simulink library "GTPR_Library"  (R2021a)
settings: Solver=VariableStepAuto  StartTime=0.0  StopTime=10.0  RelTol=1e-3
values from neighbouring files (symbols this model uses):
  aA = 0.5    [SimMechanics_GTPR_OpenLoop_CircularMotion_VS_ClosedLoop.m]
  aB = 0.5    [SimMechanics_GTPR_OpenLoop_CircularMotion_VS_ClosedLoop.m]
  aC = 0.5    [SimMechanics_GTPR_OpenLoop_CircularMotion_VS_ClosedLoop.m]
  alphaAB = deg2rad(120)    [SimMechanics_GTPR_OpenLoop_CircularMotion_VS_ClosedLoop.m]
  alphaAC = deg2rad(240)    [SimMechanics_GTPR_OpenLoop_CircularMotion_VS_ClosedLoop.m]
  eA = 0.28    [SimMechanics_GTPR_OpenLoop_CircularMotion_VS_ClosedLoop.m]
  eB = 0.28    [SimMechanics_GTPR_OpenLoop_CircularMotion_VS_ClosedLoop.m]
  eC = 0.28    [SimMechanics_GTPR_OpenLoop_CircularMotion_VS_ClosedLoop.m]
  g = -9.81    [SimMechanics_GTPR_OpenLoop_CircularMotion_VS_ClosedLoop.m]
  ILA = zeros(3)    [SimMechanics_GTPR_OpenLoop_CircularMotion_VS_ClosedLoop.m]
  IlA = zeros(3)    [SimMechanics_GTPR_OpenLoop_CircularMotion_VS_ClosedLoop.m]
  ILB = zeros(3)    [SimMechanics_GTPR_OpenLoop_CircularMotion_VS_ClosedLoop.m]
  IlB = zeros(3)    [SimMechanics_GTPR_OpenLoop_CircularMotion_VS_ClosedLoop.m]
  ILC = zeros(3)    [SimMechanics_GTPR_OpenLoop_CircularMotion_VS_ClosedLoop.m]
  IlC = zeros(3)    [SimMechanics_GTPR_OpenLoop_CircularMotion_VS_ClosedLoop.m]
  LA = 0.57    [SimMechanics_GTPR_OpenLoop_CircularMotion_VS_ClosedLoop.m]
  lA = 0.9    [SimMechanics_GTPR_OpenLoop_CircularMotion_VS_ClosedLoop.m]
  LB = 0.57    [SimMechanics_GTPR_OpenLoop_CircularMotion_VS_ClosedLoop.m]
  lB = 0.9    [SimMechanics_GTPR_OpenLoop_CircularMotion_VS_ClosedLoop.m]
  LC = 0.57    [SimMechanics_GTPR_OpenLoop_CircularMotion_VS_ClosedLoop.m]
  lC = 0.9    [SimMechanics_GTPR_OpenLoop_CircularMotion_VS_ClosedLoop.m]
  m_unaccounted = 1e-16    [SimMechanics_GTPR_OpenLoop_CircularMotion_VS_ClosedLoop.m]
  mLA = density_upperArm*VLA    (= 1.4415197891)    [SimMechanics_GTPR_OpenLoop_CircularMotion_VS_ClosedLoop.m]
  mlA = density_LowerArm*VlA    (= 0.190851753706)    [SimMechanics_GTPR_OpenLoop_CircularMotion_VS_ClosedLoop.m]
  mLB = density_upperArm*VLB    (= 1.4415197891)    [SimMechanics_GTPR_OpenLoop_CircularMotion_VS_ClosedLoop.m]
  mlB = density_LowerArm*VlB    (= 0.190851753706)    [SimMechanics_GTPR_OpenLoop_CircularMotion_VS_ClosedLoop.m]
  mLC = density_upperArm*VLC    (= 1.4415197891)    [SimMechanics_GTPR_OpenLoop_CircularMotion_VS_ClosedLoop.m]
  mlC = density_LowerArm*VlC    (= 0.190851753706)    [SimMechanics_GTPR_OpenLoop_CircularMotion_VS_ClosedLoop.m]
  mTCP = density_workTriangle * VTCP    [SimMechanics_GTPR_OpenLoop_CircularMotion_VS_ClosedLoop.m]
undefined symbols (not defined in the file or in its folder): dq1, dq2, dq3, q1, q2, q3, X, Y, Z
libraries: sm_lib x83, $bdroot x31, nesl_utility x24
(part 1 of 8)
settings Model: Creator=szucs  LastModifiedBy=szucs

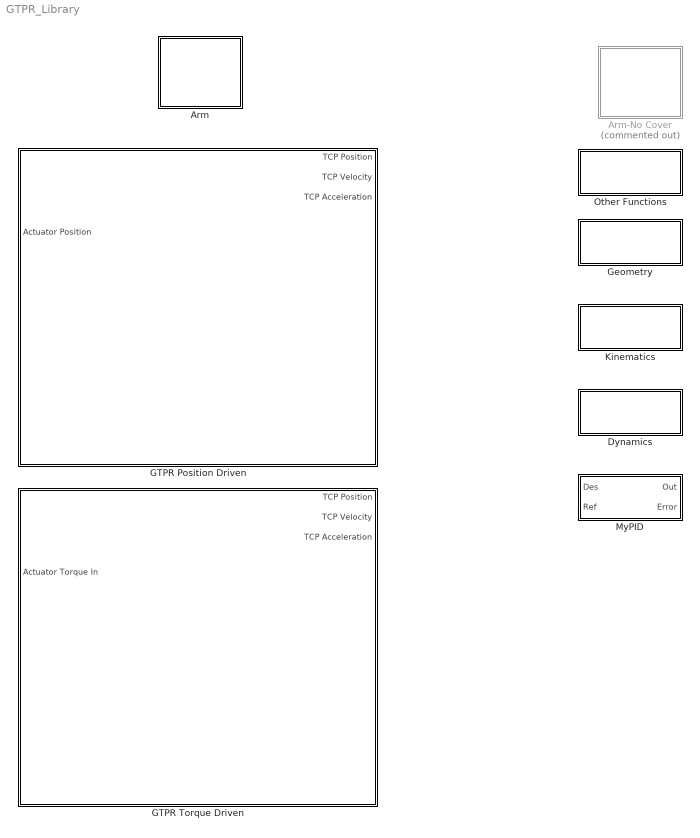
== system GTPR_Library ==
  Arm : Subsystem  mask(Delta Robot Arm){Lupper=1, RLupper=0.05, l=1, Rl=0.05, R1=0.1, L3=0.15, R2=0.05, mLupper=1, ml=1, mlink=1e-16, mTCP=0, CoverColor=[1 1 1], IL_xx=0, IL_xy=0, IL_xz=0, IL_yy=0, IL_yz=0, IL_zz=0, I_Lower_xx=0, I_Lower_xy=0, I_Lower_xz=0, I_Lower_yy=0, I_Lower_yz=0, I_Lower_zz=0}
      mask prompts: Lupper "Upper Arm Length [m]"; RLupper "Upper Arm Radius [m]"; l "Lower Arm Length [m]"; Rl "Lower Arm Radius [m]"; R1 "Joint Cover Radius [m]"; L3 "Link Length [m]"; R2 "Link Radius [m]"; mLupper "Upper Arm Mass [kg]"; ml "Lower Arm Mass [kg]"; mlink "Link Mass [kg]"; mTCP "TCP Mass [kg]"; CoverColor "Cover Color [R, G, B]"
      mask DialogControl ParameterGroupVar Prompt: Geometry
      mask DialogControl Container4 Prompt: Dimensions
      mask DialogControl Container6 Prompt: Weights
      mask DialogControl Container7 Prompt: Color
      mask DialogControl Container8 Prompt: Inertias
      mask DialogControl Container9 Prompt: Upper Arm
      mask DialogControl Container9_copy Prompt: Upper Arm
      mask Display: image(fullfile(matlabroot,'toolbox','physmod','sm','smdemos','pick_and_place_robot','images','sm_delta_robot_lib_arm.png'));
  Arm-No Cover : Subsystem  Commented=on  mask(Delta Robot Arm){Lupper=1, RLupper=0.05, l=1, Rl=0.05, R1=0.1, L3=0.15, R2=0.05, mLupper=1, ml=1, mlink=1e-16, mTCP=0, CoverColor=[1 1 1]}
      mask prompts: Lupper "Upper Arm Length [m]"; RLupper "Upper Arm Radius [m]"; l "Lower Arm Length [m]"; Rl "Lower Arm Radius [m]"; R1 "Joint Cover Radius [m]"; L3 "Link Length [m]"; R2 "Link Radius [m]"; mLupper "Upper Arm Mass [kg]"; ml "Lower Arm Mass [kg]"; mlink "Link Mass [kg]"; mTCP "TCP Mass [kg]"; CoverColor "Cover Color [R, G, B]"
      mask DialogControl ParameterGroupVar Prompt: Geometry
      mask DialogControl Container4 Prompt: Dimensions
      mask DialogControl Container6 Prompt: Weights
      mask DialogControl Container7 Prompt: Color
      mask Display: image(fullfile(matlabroot,'toolbox','physmod','sm','smdemos','pick_and_place_robot','images','sm_delta_robot_lib_arm.png'));
  Dynamics : Subsystem
  GTPR Position Driven : Subsystem  mask(Generalized Triangle Parallel Robot){LengthUpperA=LA, LengthLowerA=lA, LengthLinkA=0.1, RadiusUpperA=0.01, RadiusLowerA=0.01, RadiusLinkA=0.01, RadiusCoverA=0.02, MassUpperA=mLA, MassLowerA=mlA, MassLinkA=m_unaccounted, ColorA=[1, 0, 0], LengthUpperB=LB, LengthLowerB=lB, LengthLinkB=0.1, RadiusUpperB=0.01, RadiusLowerB=0.01, RadiusLinkB=0.01, RadiusCoverB=0.02, MassUpperB=mLB, MassLowerB=mlB, MassLinkB=m_unaccounted, ColorB=[0, 1, 0], LengthUpperC=LC, LengthLowerC=lC, LengthLinkC=0.1, RadiusUpperC=0.01, RadiusLowerC=0.01, RadiusLinkC=0.01, RadiusCoverC=0.02, MassUpperC=mLC, MassLowerC=mlC, MassLinkC=m_unaccounted, ColorC=[0, 0, 1], DistBaseA=aA, DistBaseB=aB, DistBaseC=aC, Rtop=max([aA, aB, aC]), DistWorkA=eA, DistWorkB=eB, DistWorkC=eC, MassTCP=mTCP, Rbot=max([eA, eB, eC]), NoOfSides=6, alphaAB=alphaAB, alphaAC=alphaAC}
      mask prompts: LengthUpperA "Upper Arm"; LengthLowerA "Lower Arm"; LengthLinkA "Link"; RadiusUpperA "Upper Arm"; RadiusLowerA "Lower Arm"; RadiusLinkA "Link"; RadiusCoverA "Cover"; MassUpperA "Upper Arm"; MassLowerA "Lower Arm"; MassLinkA "Link"; ColorA "Cover Color"; LengthUpperB "Upper Arm"; LengthLowerB "Lower Arm"; LengthLinkB "Link"; RadiusUpperB "Upper Arm"; RadiusLowerB "Lower Arm"; RadiusLinkB "Link"; RadiusCoverB "Cover"; MassUpperB "Upper Arm"; MassLowerB "Lower Arm"; MassLinkB "Link"; ColorB "Cover Color"; LengthUpperC "Upper Arm"; LengthLowerC "Lower Arm"; LengthLinkC "Link"; RadiusUpperC "Upper Arm"; RadiusLowerC "Lower Arm"; RadiusLinkC "Link"; RadiusCoverC "Cover"; MassUpperC "Upper Arm"; MassLowerC "Lower Arm"; MassLinkC "Link"; ColorC "Cover Color"; DistBaseA "Joint OA1 Distance [m]"; DistBaseB "Joint OB1 Distance [m]"; DistBaseC "Joint OC1 Distance [m]"; Rtop "Radius [m]"; DistWorkA "Joint TCPA3 Distance [m]"; DistWorkB "Joint TCPB3 Distance [m]"; DistWorkC "Joint TCPC3 Distance [m]"; MassTCP "Mass [kg]"; Rbot "Radius [m]"; NoOfSides "Number of Sides"; alphaAB "Angle between arms A and B [rad]"; alphaAC "Angle between arms A and C [rad]"
      mask DialogControl Container4 Prompt: Arm A
      mask DialogControl Container9 Prompt: Lengths [m]
      mask DialogControl Container10 Prompt: Radii [m]
      mask DialogControl Container11 Prompt: Masses [kg]
      mask DialogControl Container12 Prompt: Color
      mask DialogControl Container4_copy Prompt: Arm B
      mask DialogControl Container9_copy Prompt: Lengths [m]
      mask DialogControl Container10_copy Prompt: Radii [m]
      mask DialogControl Container11_copy Prompt: Masses [kg]
      mask DialogControl Container12_copy Prompt: Color
      mask DialogControl Container4_copy_copy Prompt: Arm C
      mask DialogControl Container9_copy_copy Prompt: Lengths [m]
      mask DialogControl Container10_copy_copy Prompt: Radii [m]
      mask DialogControl Container11_copy_copy Prompt: Masses [kg]
      mask DialogControl Container12_copy_copy Prompt: Color
      mask DialogControl Container25 Prompt: "Triangles" Parameters
      mask DialogControl Container27 Prompt: Base "Triangle"
      mask DialogControl Container27_copy Prompt: Work "Triangle"
  GTPR Torque Driven : Subsystem  mask(Generalized Triangle Parallel Robot){q1=q1, q2=q2, q3=q3, dq1=dq1, dq2=dq2, dq3=dq3, LengthUpperA=LA, LengthLowerA=lA, LengthLinkA=0.1, RadiusUpperA=0.01, RadiusLowerA=0.01, RadiusLinkA=0.01, RadiusCoverA=0.02, MassUpperA=mLA, MassLowerA=mlA, MassLinkA=m_unaccounted, ColorA=[1, 0, 0], IA_Upper_xx=ILA(1,1), IA_Upper_xy=ILA(1,2), IA_Upper_xz=ILA(1,3), IA_Upper_yy=ILA(2,2), IA_Upper_yz=ILA(2,3), IA_Upper_zz=ILA(3,3), IA_Lower_xx=IlA(1,1), IA_Lower_xy=IlA(1,2), IA_Lower_xz=IlA(1,3), IA_Lower_yy=IlA(2,2), IA_Lower_yz=IlA(2,3), IA_Lower_zz=IlA(3,3), LengthUpperB=LB, LengthLowerB=lB, LengthLinkB=0.1, RadiusUpperB=0.01, RadiusLowerB=0.01, RadiusLinkB=0.01, RadiusCoverB=0.02, MassUpperB=mLB, MassLowerB=mlB, MassLinkB=m_unaccounted, ColorB=[0, 1, 0], IB_Upper_xx=ILB(1,1), IB_Upper_xy=ILB(1,2), IB_Upper_xz=ILB(1,3), IB_Upper_yy=ILB(2,2), IB_Upper_yz=ILB(2,3), IB_Upper_zz=ILB(3,3), IB_Lower_xx=IlB(1,1), IB_Lower_xy=IlB(1,2), IB_Lower_xz=IlB(1,3), IB_Lower_yy=IlB(2,2), IB_Lower_yz=IlB(2,3), IB_Lower_zz=IlB(3,3), LengthUpperC=LC, LengthLowerC=lC, LengthLinkC=0.1, RadiusUpperC=0.01, RadiusLowerC=0.01, RadiusLinkC=0.01, RadiusCoverC=0.02, MassUpperC=mLC, MassLowerC=mlC, MassLinkC=m_unaccounted, ColorC=[0, 0, 1], IC_Upper_xx=ILC(1,1), IC_Upper_xy=ILC(1,2), IC_Upper_xz=ILC(1,3), IC_Upper_yy=ILC(2,2), IC_Upper_yz=ILC(2,3), IC_Upper_zz=ILC(3,3), IC_Lower_xx=IlC(1,1), IC_Lower_xy=IlC(1,2), IC_Lower_xz=IlC(1,3), IC_Lower_yy=IlC(2,2), IC_Lower_yz=IlC(2,3), IC_Lower_zz=IlC(3,3), DistBaseA=aA, DistBaseB=aB, DistBaseC=aC, Rtop=max([aA, aB, aC]), DistWorkA=eA, DistWorkB=eB, DistWorkC=eC, MassTCP=mTCP, Rbot=max([eA, eB, eC]), NoOfSides=6, alphaAB=alphaAB, alphaAC=alphaAC}
      mask prompts: q1 "Arm A Position [rad]"; q2 "Arm B Position [rad]"; q3 "Arm C Position [rad]"; dq1 "Arm A Angular Velocity [rad/s]"; dq2 "Arm B Angular Velocity [rad/s]"; dq3 "Arm C Angular Velocity [rad/s]"; LengthUpperA "Upper Arm"; LengthLowerA "Lower Arm"; LengthLinkA "Link"; RadiusUpperA "Upper Arm"; RadiusLowerA "Lower Arm"; RadiusLinkA "Link"; RadiusCoverA "Cover"; MassUpperA "Upper Arm"; MassLowerA "Lower Arm"; MassLinkA "Link"; ColorA "Cover Color"; IA_Upper_xx "I_Upper_xx"; IA_Upper_xy "I_Upper_xy"; IA_Upper_xz "I_Upper_xz"; IA_Upper_yy "I_Upper_yy"; IA_Upper_yz "I_Upper_yz"; IA_Upper_zz "I_Upper_zz"; IA_Lower_xx "I_Lower_xx"; IA_Lower_xy "I_Lower_xy"; IA_Lower_xz "I_Lower_xz"; IA_Lower_yy "I_Lower_yy"; IA_Lower_yz "I_Lower_yz"; IA_Lower_zz "I_Lower_zz"; LengthUpperB "Upper Arm"; LengthLowerB "Lower Arm"; LengthLinkB "Link"; RadiusUpperB "Upper Arm"; RadiusLowerB "Lower Arm"; RadiusLinkB "Link"; RadiusCoverB "Cover"; MassUpperB "Upper Arm"; MassLowerB "Lower Arm"; MassLinkB "Link"; ColorB "Cover Color"; IB_Upper_xx "I_Upper_xx"; IB_Upper_xy "I_Upper_xy"; IB_Upper_xz "I_Upper_xz"; IB_Upper_yy "I_Upper_yy"; IB_Upper_yz "I_Upper_yz"; IB_Upper_zz "I_Upper_zz"; IB_Lower_xx "I_Lower_xx"; IB_Lower_xy "I_Lower_xy"; IB_Lower_xz "I_Lower_xz"; IB_Lower_yy "I_Lower_yy"; IB_Lower_yz "I_Lower_yz"; IB_Lower_zz "I_Lower_zz"; LengthUpperC "Upper Arm"; LengthLowerC "Lower Arm"; LengthLinkC "Link"; RadiusUpperC "Upper Arm"; RadiusLowerC "Lower Arm"; RadiusLinkC "Link"; RadiusCoverC "Cover"; MassUpperC "Upper Arm"; MassLowerC "Lower Arm"; MassLinkC "Link"; ColorC "Cover Color"; IC_Upper_xx "I_Upper_xx"; IC_Upper_xy "I_Upper_xy"; IC_Upper_xz "I_Upper_xz"; IC_Upper_yy "I_Upper_yy"; IC_Upper_yz "I_Upper_yz"; IC_Upper_zz "I_Upper_zz"; IC_Lower_xx "I_Lower_xx"; IC_Lower_xy "I_Lower_xy"; IC_Lower_xz "I_Lower_xz"; IC_Lower_yy "I_Lower_yy"; IC_Lower_yz "I_Lower_yz"; IC_Lower_zz "I_Lower_zz"; DistBaseA "Joint OA1 Distance [m]"; DistBaseB "Joint OB1 Distance [m]"; DistBaseC "Joint OC1 Distance [m]"; Rtop "Radius [m]"; DistWorkA "Joint TCPA3 Distance [m]"; DistWorkB "Joint TCPB3 Distance [m]"; DistWorkC "Joint TCPC3 Distance [m]"; MassTCP "Mass [kg]"; Rbot "Radius [m]"; NoOfSides "Number of Sides"; alphaAB "Angle between arms A and B [rad]"; alphaAC "Angle between arms A and C [rad]"
      mask DialogControl Container32 Prompt: Initial Parameters
      mask DialogControl Container4 Prompt: Arm A
      mask DialogControl Container9 Prompt: Lengths [m]
      mask DialogControl Container10 Prompt: Radii [m]
      mask DialogControl Container11 Prompt: Masses [kg]
      mask DialogControl Container12 Prompt: Color
      mask DialogControl Container29 Prompt: Inertia Parameters
      mask DialogControl Container30 Prompt: Upper Arm
      mask DialogControl Container30_copy Prompt: Lower Arm
      mask DialogControl Container4_copy Prompt: Arm B
      mask DialogControl Container9_copy Prompt: Lengths [m]
      mask DialogControl Container10_copy Prompt: Radii [m]
      mask DialogControl Container11_copy Prompt: Masses [kg]
      mask DialogControl Container12_copy Prompt: Color
      mask DialogControl Container29_copy Prompt: Inertia Parameters
      mask DialogControl Container30_copy_copy Prompt: Upper Arm
      mask DialogControl Container30_copy_copy_copy Prompt: Lower Arm
      mask DialogControl Container4_copy_copy Prompt: Arm C
      mask DialogControl Container9_copy_copy Prompt: Lengths [m]
      mask DialogControl Container10_copy_copy Prompt: Radii [m]
      mask DialogControl Container11_copy_copy Prompt: Masses [kg]
      mask DialogControl Container12_copy_copy Prompt: Color
      mask DialogControl Container29_copy_copy Prompt: Inertia Parameters
      mask DialogControl Container30_copy_copy_copy_copy Prompt: Upper Arm
      mask DialogControl Container30_copy_copy_copy_copy_copy Prompt: Lower Arm
      mask DialogControl Container25 Prompt: "Triangles" Parameters
      mask DialogControl Container27 Prompt: Base "Triangle"
      mask DialogControl Container27_copy Prompt: Work "Triangle"
  Geometry : Subsystem
  Kinematics : Subsystem
  MyPID : Subsystem  mask{P=0, I=0, D=0}
  Other Functions : Subsystem

== system GTPR_Library/Arm ==
  Elbow Joint : sm_lib/Joints/Revolute Joint  JointMode=Normal  SenseConstraintForce=off  SenseConstraintForceX=off  SenseConstraintForceY=off  SenseConstraintForceZ=off  SenseConstraintTorque=off  SenseConstraintTorqueX=off  SenseConstraintTorqueY=off  SenseConstraintTorqueZ=off  SenseTotalForce=off  SenseTotalForceX=off  SenseTotalForceY=off  SenseTotalForceZ=off  SenseTotalTorque=off  SenseTotalTorqueX=off  SenseTotalTorqueY=off  SenseTotalTorqueZ=off  CompositeWrenchDir=FollowerOnBase  CompositeWrenchFrame=BaseFrame  EquilibriumPosition=0  EquilibriumPositionUnits=deg  SpringStiffness=0  SpringStiffnessUnits=N*m/deg  DampingCoefficient=0  DampingCoefficientUnits=N*m/(deg/s)  TorqueActuationMode=NoTorque  MotionActuationMode=ComputedMotion  SensePosition=off  SenseVelocity=off  SenseAcceleration=off  SenseTorqueForce=off  SenseLowerLimitTorqueForce=off  SenseUpperLimitTorqueForce=off  LowerLimitSpecify=off  LowerLimitBound=-90  LowerLimitBoundUnits=deg  LowerLimitStiffness=1e4  LowerLimitStiffnessUnits=N*m/deg  LowerLimitDamping=10  LowerLimitDampingUnits=N*m/(deg/s)  LowerLimitTransitionRegionWidth=0.1  LowerLimitTransitionRegionWidthUnits=deg  UpperLimitSpecify=off  UpperLimitBound=90  UpperLimitBoundUnits=deg  UpperLimitStiffness=1e4  UpperLimitStiffnessUnits=N*m/deg  UpperLimitDamping=10  UpperLimitDampingUnits=N*m/(deg/s)  UpperLimitTransitionRegionWidth=0.1  UpperLimitTransitionRegionWidthUnits=deg  PositionTargetSpecify=off  PositionTargetPriority=High  PositionTargetValue=0  PositionTargetValueUnits=deg  VelocityTargetSpecify=off  VelocityTargetPriority=High  VelocityTargetValue=0  VelocityTargetValueUnits=deg/s
  Lower Arm : Subsystem
  Upper Arm : Subsystem
  Top : PMIOPort  Side=Left
  Bot : PMIOPort  Port=2  Side=Right
  connections:
  Lower Arm/RConn1 -- Bot/RConn1
  Lower Arm/LConn1 -- Elbow Joint/RConn1
  Top/RConn1 -- Upper Arm/LConn1
  Upper Arm/RConn1 -- Elbow Joint/LConn1

== system GTPR_Library/Arm-No Cover ==
  Elbow Joint : sm_lib/Joints/Revolute Joint  JointMode=Normal  SenseConstraintForce=off  SenseConstraintForceX=off  SenseConstraintForceY=off  SenseConstraintForceZ=off  SenseConstraintTorque=off  SenseConstraintTorqueX=off  SenseConstraintTorqueY=off  SenseConstraintTorqueZ=off  SenseTotalForce=off  SenseTotalForceX=off  SenseTotalForceY=off  SenseTotalForceZ=off  SenseTotalTorque=off  SenseTotalTorqueX=off  SenseTotalTorqueY=off  SenseTotalTorqueZ=off  CompositeWrenchDir=FollowerOnBase  CompositeWrenchFrame=BaseFrame  EquilibriumPosition=0  EquilibriumPositionUnits=deg  SpringStiffness=0  SpringStiffnessUnits=N*m/deg  DampingCoefficient=0  DampingCoefficientUnits=N*m/(deg/s)  TorqueActuationMode=NoTorque  MotionActuationMode=ComputedMotion  SensePosition=off  SenseVelocity=off  SenseAcceleration=off  SenseTorqueForce=off  SenseLowerLimitTorqueForce=off  SenseUpperLimitTorqueForce=off  LowerLimitSpecify=off  LowerLimitBound=-90  LowerLimitBoundUnits=deg  LowerLimitStiffness=1e4  LowerLimitStiffnessUnits=N*m/deg  LowerLimitDamping=10  LowerLimitDampingUnits=N*m/(deg/s)  LowerLimitTransitionRegionWidth=0.1  LowerLimitTransitionRegionWidthUnits=deg  UpperLimitSpecify=off  UpperLimitBound=90  UpperLimitBoundUnits=deg  UpperLimitStiffness=1e4  UpperLimitStiffnessUnits=N*m/deg  UpperLimitDamping=10  UpperLimitDampingUnits=N*m/(deg/s)  UpperLimitTransitionRegionWidth=0.1  UpperLimitTransitionRegionWidthUnits=deg  PositionTargetSpecify=off  PositionTargetPriority=High  PositionTargetValue=0  PositionTargetValueUnits=deg  VelocityTargetSpecify=off  VelocityTargetPriority=High  VelocityTargetValue=0  VelocityTargetValueUnits=deg/s
  Lower Arm : Subsystem
  Upper Arm : Subsystem
  Top : PMIOPort  Side=Left
  Bot : PMIOPort  Port=2  Side=Right
  connections:
  Lower Arm/RConn1 -- Bot/RConn1
  Lower Arm/LConn1 -- Elbow Joint/RConn1
  Top/RConn1 -- Upper Arm/LConn1
  Upper Arm/RConn1 -- Elbow Joint/LConn1

== system GTPR_Library/Dynamics ==
  DynamicEquations : Subsystem  mask{aA=aA, aB=aB, aC=aC, alphaAB=alphaAB, alphaAC=alphaAC, LAu=LA, LBu=LB, LCu=LC, lA=lA, lB=lB, lC=lC, eA=eA, eB=eB, eC=eC, ILAu=ILA, ILBu=ILB, ILCu=ILC, IlA=IlA, IlB=IlB, IlC=IlC, g=g, mLAu=mLA, mLBu=mLB, mLCu=mLC, mlA=mlA, mlB=mlB, mlC=mlC, mTCP=mTCP}
      mask prompts: LAu "LA"; LBu "LB"; LCu "LC"; ILAu "ILA"; ILBu "ILB"; ILCu "ILC"; mLAu "mLA"; mLBu "mLB"; mLCu "mLC"
  Initialize Dynamic Equations : Subsystem  Commented=on  mask{filepath="C:\Git\PhD\Matlab\GTPR\Engine\DynamicEquations.m"}
      mask prompts: filepath "Path to "DynamicEquations.m""
  Inverse Dynamics : Subsystem  Commented=on

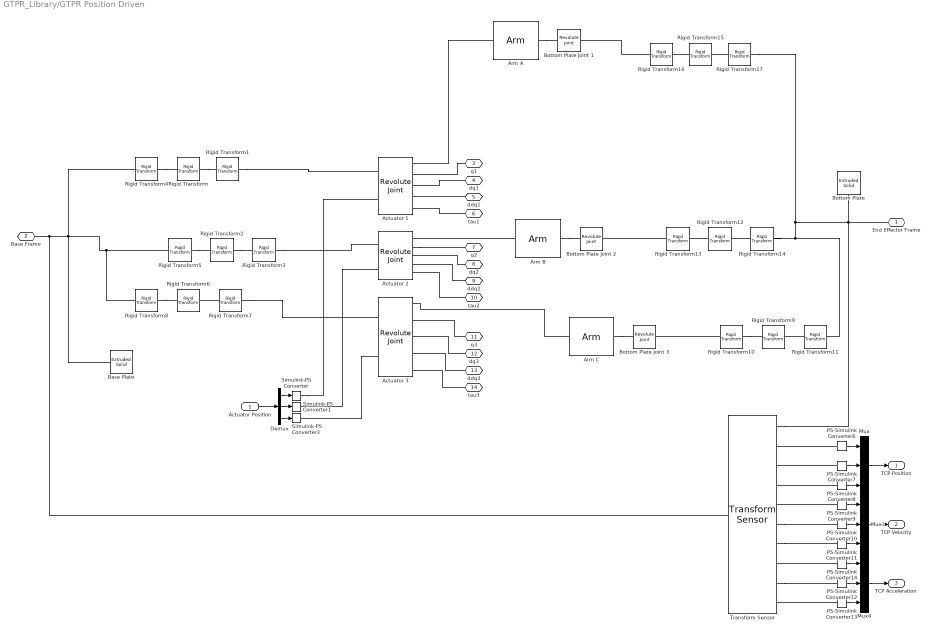
== system GTPR_Library/GTPR Position Driven ==
  Actuator Position : Inport
  Actuator 1 : sm_lib/Joints/Revolute Joint  JointMode=Normal  SenseConstraintForce=off  SenseConstraintForceX=off  SenseConstraintForceY=off  SenseConstraintForceZ=off  SenseConstraintTorque=off  SenseConstraintTorqueX=off  SenseConstraintTorqueY=off  SenseConstraintTorqueZ=off  SenseTotalForce=off  SenseTotalForceX=off  SenseTotalForceY=off  SenseTotalForceZ=off  SenseTotalTorque=off  SenseTotalTorqueX=off  SenseTotalTorqueY=off  SenseTotalTorqueZ=off  CompositeWrenchDir=FollowerOnBase  CompositeWrenchFrame=BaseFrame  EquilibriumPosition=0  EquilibriumPositionUnits=deg  SpringStiffness=0  SpringStiffnessUnits=N*m/deg  DampingCoefficient=0  DampingCoefficientUnits=N*m/(deg/s)  TorqueActuationMode=ComputedTorque  MotionActuationMode=InputMotion  SensePosition=on  SenseVelocity=on  SenseAcceleration=on  SenseTorqueForce=on  SenseLowerLimitTorqueForce=off  SenseUpperLimitTorqueForce=off  LowerLimitSpecify=off  LowerLimitBound=-10  LowerLimitBoundUnits=deg  LowerLimitStiffness=1e4  LowerLimitStiffnessUnits=N*m/deg  LowerLimitDamping=10  LowerLimitDampingUnits=N*m/(deg/s)  LowerLimitTransitionRegionWidth=0.1  LowerLimitTransitionRegionWidthUnits=deg  UpperLimitSpecify=off  UpperLimitBound=90  UpperLimitBoundUnits=deg  UpperLimitStiffness=1e4  UpperLimitStiffnessUnits=N*m/deg  UpperLimitDamping=10  UpperLimitDampingUnits=N*m/(deg/s)  UpperLimitTransitionRegionWidth=0.1  UpperLimitTransitionRegionWidthUnits=deg  PositionTargetSpecify=on  PositionTargetPriority=High  PositionTargetValue=q1  PositionTargetValueUnits=rad  VelocityTargetSpecify=on  VelocityTargetPriority=High  VelocityTargetValue=dq1  VelocityTargetValueUnits=rad/s
  Actuator 2 : sm_lib/Joints/Revolute Joint  JointMode=Normal  SenseConstraintForce=off  SenseConstraintForceX=off  SenseConstraintForceY=off  SenseConstraintForceZ=off  SenseConstraintTorque=off  SenseConstraintTorqueX=off  SenseConstraintTorqueY=off  SenseConstraintTorqueZ=off  SenseTotalForce=off  SenseTotalForceX=off  SenseTotalForceY=off  SenseTotalForceZ=off  SenseTotalTorque=off  SenseTotalTorqueX=off  SenseTotalTorqueY=off  SenseTotalTorqueZ=off  CompositeWrenchDir=FollowerOnBase  CompositeWrenchFrame=BaseFrame  EquilibriumPosition=0  EquilibriumPositionUnits=deg  SpringStiffness=0  SpringStiffnessUnits=N*m/deg  DampingCoefficient=0  DampingCoefficientUnits=N*m/(deg/s)  TorqueActuationMode=ComputedTorque  MotionActuationMode=InputMotion  SensePosition=on  SenseVelocity=on  SenseAcceleration=on  SenseTorqueForce=on  SenseLowerLimitTorqueForce=off  SenseUpperLimitTorqueForce=off  LowerLimitSpecify=off  LowerLimitBound=-10  LowerLimitBoundUnits=deg  LowerLimitStiffness=1e4  LowerLimitStiffnessUnits=N*m/deg  LowerLimitDamping=10  LowerLimitDampingUnits=N*m/(deg/s)  LowerLimitTransitionRegionWidth=0.1  LowerLimitTransitionRegionWidthUnits=deg  UpperLimitSpecify=off  UpperLimitBound=90  UpperLimitBoundUnits=deg  UpperLimitStiffness=1e4  UpperLimitStiffnessUnits=N*m/deg  UpperLimitDamping=10  UpperLimitDampingUnits=N*m/(deg/s)  UpperLimitTransitionRegionWidth=0.1  UpperLimitTransitionRegionWidthUnits=deg  PositionTargetSpecify=on  PositionTargetPriority=High  PositionTargetValue=q2  PositionTargetValueUnits=rad  VelocityTargetSpecify=on  VelocityTargetPriority=High  VelocityTargetValue=dq2  VelocityTargetValueUnits=rad/s
  Actuator 3 : sm_lib/Joints/Revolute Joint  JointMode=Normal  SenseConstraintForce=off  SenseConstraintForceX=off  SenseConstraintForceY=off  SenseConstraintForceZ=off  SenseConstraintTorque=off  SenseConstraintTorqueX=off  SenseConstraintTorqueY=off  SenseConstraintTorqueZ=off  SenseTotalForce=off  SenseTotalForceX=off  SenseTotalForceY=off  SenseTotalForceZ=off  SenseTotalTorque=off  SenseTotalTorqueX=off  SenseTotalTorqueY=off  SenseTotalTorqueZ=off  CompositeWrenchDir=FollowerOnBase  CompositeWrenchFrame=BaseFrame  EquilibriumPosition=0  EquilibriumPositionUnits=deg  SpringStiffness=0  SpringStiffnessUnits=N*m/deg  DampingCoefficient=0  DampingCoefficientUnits=N*m/(deg/s)  TorqueActuationMode=ComputedTorque  MotionActuationMode=InputMotion  SensePosition=on  SenseVelocity=on  SenseAcceleration=on  SenseTorqueForce=on  SenseLowerLimitTorqueForce=off  SenseUpperLimitTorqueForce=off  LowerLimitSpecify=off  LowerLimitBound=-10  LowerLimitBoundUnits=deg  LowerLimitStiffness=1e4  LowerLimitStiffnessUnits=N*m/deg  LowerLimitDamping=10  LowerLimitDampingUnits=N*m/(deg/s)  LowerLimitTransitionRegionWidth=0.1  LowerLimitTransitionRegionWidthUnits=deg  UpperLimitSpecify=off  UpperLimitBound=90  UpperLimitBoundUnits=deg  UpperLimitStiffness=1e4  UpperLimitStiffnessUnits=N*m/deg  UpperLimitDamping=10  UpperLimitDampingUnits=N*m/(deg/s)  UpperLimitTransitionRegionWidth=0.1  UpperLimitTransitionRegionWidthUnits=deg  PositionTargetSpecify=on  PositionTargetPriority=High  PositionTargetValue=q3  PositionTargetValueUnits=rad  VelocityTargetSpecify=on  VelocityTargetPriority=High  VelocityTargetValue=dq3  VelocityTargetValueUnits=rad/s
  Arm A : $bdroot/Arm  Lupper=LengthUpperA  RLupper=RadiusUpperA  l=LengthLowerA  Rl=RadiusLowerA  R1=RadiusCoverA  L3=LengthLinkA  R2=RadiusLinkA  mLupper=MassUpperA  ml=MassLowerA  mlink=MassLinkA  mTCP=0  CoverColor=ColorA  IL_xx=0  IL_xy=0  IL_xz=0  IL_yy=0  IL_yz=0  IL_zz=0  I_Lower_xx=0  I_Lower_xy=0  I_Lower_xz=0  I_Lower_yy=0  I_Lower_yz=0  I_Lower_zz=0
  Arm B : $bdroot/Arm  Lupper=LengthUpperB  RLupper=RadiusUpperB  l=LengthLowerB  Rl=RadiusLowerB  R1=RadiusCoverB  L3=LengthLinkB  R2=RadiusLinkB  mLupper=MassUpperB  ml=MassLowerB  mlink=MassLinkB  mTCP=0  CoverColor=ColorB  IL_xx=0  IL_xy=0  IL_xz=0  IL_yy=0  IL_yz=0  IL_zz=0  I_Lower_xx=0  I_Lower_xy=0  I_Lower_xz=0  I_Lower_yy=0  I_Lower_yz=0  I_Lower_zz=0
  Arm C : $bdroot/Arm  Lupper=LengthUpperC  RLupper=RadiusUpperC  l=LengthLowerC  Rl=RadiusLowerC  R1=RadiusCoverC  L3=LengthLinkC  R2=RadiusLinkC  mLupper=MassUpperC  ml=MassLowerC  mlink=MassLinkC  mTCP=0  CoverColor=ColorC  IL_xx=0  IL_xy=0  IL_xz=0  IL_yy=0  IL_yz=0  IL_zz=0  I_Lower_xx=0  I_Lower_xy=0  I_Lower_xz=0  I_Lower_yy=0  I_Lower_yz=0  I_Lower_zz=0
  Base Plate : sm_lib/Body Elements/Extruded Solid  GraphicAmbientColor=[0.15 0.15 0.15 1.0]  BasedOnType=Density  CenterOfMass=[0 0 0]  CenterOfMassUnits=m  GraphicDiffuseColor=[0.5 0.5 0.5]  ExportConvexHullGeometry=off  ExtrusionCrossSection=[1 1; -1 1; -1 -1; 1 -1]  ExtrusionCrossSectionUnits=m  Density=1000  DensityUnits=kg/m^3  DoExposeReferenceFrame=on  GraphicEmissiveColor=[0.0 0.0 0.0 1.0]  ExportEntireGeometry=off  ExtrusionLength=Rtop/15  ExtrusionLengthUnits=m  ExtrusionType=Regular  SerializedFrames=<Frames/>  MarkerShape=Sphere  MarkerSize=10  GraphicType=FromGeometry  InertiaType=CalculateFromGeometry  Mass=1  MassUnits=kg  MomentsOfInertia=[1 1 1]  MomentsOfInertiaUnits=kg*m^2  PolygonNumSides=NoOfSides  GraphicOpacity=1.0  PolygonOuterRadius=Rtop  PolygonOuterRadiusUnits=m  ProductsOfInertia=[0 0 0]  ProductsOfInertiaUnits=kg*m^2  GraphicShininess=75  GraphicSpecularColor=[0.5 0.5 0.5 1.0]  GraphicVisPropType=SimpleVisualProperties
  Bottom Plate : sm_lib/Body Elements/Extruded Solid  GraphicAmbientColor=[0.15 0.15 0.15 1.0]  BasedOnType=Mass  CenterOfMass=[0 0 0]  CenterOfMassUnits=m  GraphicDiffuseColor=[0.5 0.5 0.5]  ExportConvexHullGeometry=off  ExtrusionCrossSection=[1 1; -1 1; -1 -1; 1 -1]  ExtrusionCrossSectionUnits=m  Density=1000  DensityUnits=kg/m^3  DoExposeReferenceFrame=on  GraphicEmissiveColor=[0.0 0.0 0.0 1.0]  ExportEntireGeometry=off  ExtrusionLength=Rbot/15  ExtrusionLengthUnits=m  ExtrusionType=Regular  SerializedFrames=<Frames/>  MarkerShape=Sphere  MarkerSize=10  GraphicType=FromGeometry  InertiaType=CalculateFromGeometry  Mass=m_unaccounted  MassUnits=kg  MomentsOfInertia=[1 1 1]  MomentsOfInertiaUnits=kg*m^2  PolygonNumSides=NoOfSides  GraphicOpacity=0.5  PolygonOuterRadius=Rbot  PolygonOuterRadiusUnits=m  ProductsOfInertia=[0 0 0]  ProductsOfInertiaUnits=kg*m^2  GraphicShininess=75  GraphicSpecularColor=[0.5 0.5 0.5 1.0]  GraphicVisPropType=SimpleVisualProperties
  Bottom Plate Joint 1 : sm_lib/Joints/Revolute Joint  JointMode=Normal  SenseConstraintForce=off  SenseConstraintForceX=off  SenseConstraintForceY=off  SenseConstraintForceZ=off  SenseConstraintTorque=off  SenseConstraintTorqueX=off  SenseConstraintTorqueY=off  SenseConstraintTorqueZ=off  SenseTotalForce=off  SenseTotalForceX=off  SenseTotalForceY=off  SenseTotalForceZ=off  SenseTotalTorque=off  SenseTotalTorqueX=off  SenseTotalTorqueY=off  SenseTotalTorqueZ=off  CompositeWrenchDir=FollowerOnBase  CompositeWrenchFrame=BaseFrame  EquilibriumPosition=0  EquilibriumPositionUnits=deg  SpringStiffness=0  SpringStiffnessUnits=N*m/deg  DampingCoefficient=0  DampingCoefficientUnits=N*m/(deg/s)  TorqueActuationMode=NoTorque  MotionActuationMode=ComputedMotion  SensePosition=off  SenseVelocity=off  SenseAcceleration=off  SenseTorqueForce=off  SenseLowerLimitTorqueForce=off  SenseUpperLimitTorqueForce=off  LowerLimitSpecify=off  LowerLimitBound=-90  LowerLimitBoundUnits=deg  LowerLimitStiffness=1e4  LowerLimitStiffnessUnits=N*m/deg  LowerLimitDamping=10  LowerLimitDampingUnits=N*m/(deg/s)  LowerLimitTransitionRegionWidth=0.1  LowerLimitTransitionRegionWidthUnits=deg  UpperLimitSpecify=off  UpperLimitBound=90  UpperLimitBoundUnits=deg  UpperLimitStiffness=1e4  UpperLimitStiffnessUnits=N*m/deg  UpperLimitDamping=10  UpperLimitDampingUnits=N*m/(deg/s)  UpperLimitTransitionRegionWidth=0.1  UpperLimitTransitionRegionWidthUnits=deg  PositionTargetSpecify=off  PositionTargetPriority=High  PositionTargetValue=0  PositionTargetValueUnits=deg  VelocityTargetSpecify=off  VelocityTargetPriority=High  VelocityTargetValue=0  VelocityTargetValueUnits=deg/s
  Bottom Plate Joint 2 : sm_lib/Joints/Revolute Joint  JointMode=Normal  SenseConstraintForce=off  SenseConstraintForceX=off  SenseConstraintForceY=off  SenseConstraintForceZ=off  SenseConstraintTorque=off  SenseConstraintTorqueX=off  SenseConstraintTorqueY=off  SenseConstraintTorqueZ=off  SenseTotalForce=off  SenseTotalForceX=off  SenseTotalForceY=off  SenseTotalForceZ=off  SenseTotalTorque=off  SenseTotalTorqueX=off  SenseTotalTorqueY=off  SenseTotalTorqueZ=off  CompositeWrenchDir=FollowerOnBase  CompositeWrenchFrame=BaseFrame  EquilibriumPosition=0  EquilibriumPositionUnits=deg  SpringStiffness=0  SpringStiffnessUnits=N*m/deg  DampingCoefficient=0  DampingCoefficientUnits=N*m/(deg/s)  TorqueActuationMode=NoTorque  MotionActuationMode=ComputedMotion  SensePosition=off  SenseVelocity=off  SenseAcceleration=off  SenseTorqueForce=off  SenseLowerLimitTorqueForce=off  SenseUpperLimitTorqueForce=off  LowerLimitSpecify=off  LowerLimitBound=-90  LowerLimitBoundUnits=deg  LowerLimitStiffness=1e4  LowerLimitStiffnessUnits=N*m/deg  LowerLimitDamping=10  LowerLimitDampingUnits=N*m/(deg/s)  LowerLimitTransitionRegionWidth=0.1  LowerLimitTransitionRegionWidthUnits=deg  UpperLimitSpecify=off  UpperLimitBound=90  UpperLimitBoundUnits=deg  UpperLimitStiffness=1e4  UpperLimitStiffnessUnits=N*m/deg  UpperLimitDamping=10  UpperLimitDampingUnits=N*m/(deg/s)  UpperLimitTransitionRegionWidth=0.1  UpperLimitTransitionRegionWidthUnits=deg  PositionTargetSpecify=off  PositionTargetPriority=High  PositionTargetValue=0  PositionTargetValueUnits=deg  VelocityTargetSpecify=off  VelocityTargetPriority=High  VelocityTargetValue=0  VelocityTargetValueUnits=deg/s
  Bottom Plate Joint 3 : sm_lib/Joints/Revolute Joint  JointMode=Normal  SenseConstraintForce=off  SenseConstraintForceX=off  SenseConstraintForceY=off  SenseConstraintForceZ=off  SenseConstraintTorque=off  SenseConstraintTorqueX=off  SenseConstraintTorqueY=off  SenseConstraintTorqueZ=off  SenseTotalForce=off  SenseTotalForceX=off  SenseTotalForceY=off  SenseTotalForceZ=off  SenseTotalTorque=off  SenseTotalTorqueX=off  SenseTotalTorqueY=off  SenseTotalTorqueZ=off  CompositeWrenchDir=FollowerOnBase  CompositeWrenchFrame=BaseFrame  EquilibriumPosition=0  EquilibriumPositionUnits=deg  SpringStiffness=0  SpringStiffnessUnits=N*m/deg  DampingCoefficient=0  DampingCoefficientUnits=N*m/(deg/s)  TorqueActuationMode=NoTorque  MotionActuationMode=ComputedMotion  SensePosition=off  SenseVelocity=off  SenseAcceleration=off  SenseTorqueForce=off  SenseLowerLimitTorqueForce=off  SenseUpperLimitTorqueForce=off  LowerLimitSpecify=off  LowerLimitBound=-90  LowerLimitBoundUnits=deg  LowerLimitStiffness=1e4  LowerLimitStiffnessUnits=N*m/deg  LowerLimitDamping=10  LowerLimitDampingUnits=N*m/(deg/s)  LowerLimitTransitionRegionWidth=0.1  LowerLimitTransitionRegionWidthUnits=deg  UpperLimitSpecify=off  UpperLimitBound=90  UpperLimitBoundUnits=deg  UpperLimitStiffness=1e4  UpperLimitStiffnessUnits=N*m/deg  UpperLimitDamping=10  UpperLimitDampingUnits=N*m/(deg/s)  UpperLimitTransitionRegionWidth=0.1  UpperLimitTransitionRegionWidthUnits=deg  PositionTargetSpecify=off  PositionTargetPriority=High  PositionTargetValue=0  PositionTargetValueUnits=deg  VelocityTargetSpecify=off  VelocityTargetPriority=High  VelocityTargetValue=0  VelocityTargetValueUnits=deg/s
  Demux : Demux  Outputs=3
  Mux : Mux  Inputs=3
  Mux3 : Mux  Inputs=3
  Mux4 : Mux  Inputs=3
  PS-Simulink Converter10 : nesl_utility/PS-Simulink Converter  PhysicalDomain=network_engine_domain  SubClassName=ps_output  LeftPortType=input  RightPortType=output  PseudoPeriodic=off  Frequencies=[]  Unit=m/s  AffineConversion=off
      settings: SourceProductBaseCode=PW,SS
  PS-Simulink Converter11 : nesl_utility/PS-Simulink Converter  PhysicalDomain=network_engine_domain  SubClassName=ps_output  LeftPortType=input  RightPortType=output  PseudoPeriodic=off  Frequencies=[]  Unit=m/s  AffineConversion=off
      settings: SourceProductBaseCode=PW,SS
  PS-Simulink Converter12 : nesl_utility/PS-Simulink Converter  PhysicalDomain=network_engine_domain  SubClassName=ps_output  LeftPortType=input  RightPortType=output  PseudoPeriodic=off  Frequencies=[]  Unit=m/s^2  AffineConversion=off
      settings: SourceProductBaseCode=PW,SS
  PS-Simulink Converter13 : nesl_utility/PS-Simulink Converter  PhysicalDomain=network_engine_domain  SubClassName=ps_output  LeftPortType=input  RightPortType=output  PseudoPeriodic=off  Frequencies=[]  Unit=m/s^2  AffineConversion=off
      settings: SourceProductBaseCode=PW,SS
  PS-Simulink Converter14 : nesl_utility/PS-Simulink Converter  PhysicalDomain=network_engine_domain  SubClassName=ps_output  LeftPortType=input  RightPortType=output  PseudoPeriodic=off  Frequencies=[]  Unit=m/s^2  AffineConversion=off
      settings: SourceProductBaseCode=PW,SS
  PS-Simulink Converter6 : nesl_utility/PS-Simulink Converter  PhysicalDomain=network_engine_domain  SubClassName=ps_output  LeftPortType=input  RightPortType=output  PseudoPeriodic=off  Frequencies=[]  Unit=m  AffineConversion=off
      settings: SourceProductBaseCode=PW,SS
  PS-Simulink Converter7 : nesl_utility/PS-Simulink Converter  PhysicalDomain=network_engine_domain  SubClassName=ps_output  LeftPortType=input  RightPortType=output  PseudoPeriodic=off  Frequencies=[]  Unit=m  AffineConversion=off
      settings: SourceProductBaseCode=PW,SS
  PS-Simulink Converter8 : nesl_utility/PS-Simulink Converter  PhysicalDomain=network_engine_domain  SubClassName=ps_output  LeftPortType=input  RightPortType=output  PseudoPeriodic=off  Frequencies=[]  Unit=m  AffineConversion=off
      settings: SourceProductBaseCode=PW,SS
  PS-Simulink Converter9 : nesl_utility/PS-Simulink Converter  PhysicalDomain=network_engine_domain  SubClassName=ps_output  LeftPortType=input  RightPortType=output  PseudoPeriodic=off  Frequencies=[]  Unit=m/s  AffineConversion=off
      settings: SourceProductBaseCode=PW,SS
  Rigid Transform{,2,6,9,12,15} (6 alike) : sm_lib/Frames and Transforms/Rigid Transform  TranslationMethod=None  TranslationStandardOffset=0  TranslationLengthUnit=m  TranslationStandardAxis=+Z  TranslationCartesianOffset=[0 -aA 0]  TranslationROffset=0  TranslationROffsetUnits=m  TranslationZOffset=0  TranslationZOffsetUnits=m  TranslationThetaOffset=0  TranslationThetaOffsetUnits=deg  RotationMethod=StandardAxis  RotationAngleUnits=deg  RotationStandardAxis=+X  RotationAngle=-90  RotationArbitraryAxis=[0 0 1]  FollAlignAxisA=+X  BaseAlignAxisA=+Y  FollAlignAxisB=+Y  BaseAlignAxisB=+Z  RotationSequenceAxes=FollowerAxes  RotationSequence=XYX  RotationSequenceAngles=[0 0 0]  RotationSequenceAnglesUnits=deg  RotationMatrix=[1 0 0; 0 1 0; 0 0 1]
  Rigid Transform1 : sm_lib/Frames and Transforms/Rigid Transform  TranslationMethod=None  TranslationStandardOffset=0  TranslationLengthUnit=m  TranslationStandardAxis=+Z  TranslationCartesianOffset=[0 0 0]  TranslationROffset=0  TranslationROffsetUnits=m  TranslationZOffset=0  TranslationZOffsetUnits=m  TranslationThetaOffset=0  TranslationThetaOffsetUnits=deg  RotationMethod=StandardAxis  RotationAngleUnits=deg  RotationStandardAxis=+Y  RotationAngle=90  RotationArbitraryAxis=[0 0 1]  FollAlignAxisA=+X  BaseAlignAxisA=+Z  FollAlignAxisB=+Z  BaseAlignAxisB=+X  RotationSequenceAxes=FollowerAxes  RotationSequence=XYX  RotationSequenceAngles=[0 0 0]  RotationSequenceAnglesUnits=deg  RotationMatrix=[1 0 0; 0 1 0; 0 0 1]
  Rigid Transform10 : sm_lib/Frames and Transforms/Rigid Transform  TranslationMethod=None  TranslationStandardOffset=0  TranslationLengthUnit=m  TranslationStandardAxis=+Z  TranslationCartesianOffset=[0 0 0]  TranslationROffset=0  TranslationROffsetUnits=m  TranslationZOffset=0  TranslationZOffsetUnits=m  TranslationThetaOffset=0  TranslationThetaOffsetUnits=deg  RotationMethod=StandardAxis  RotationAngleUnits=rad  RotationStandardAxis=+Y  RotationAngle=(pi/2) + alphaAC  RotationArbitraryAxis=[0 0 1]  FollAlignAxisA=+X  BaseAlignAxisA=+Z  FollAlignAxisB=+Z  BaseAlignAxisB=+X  RotationSequenceAxes=FollowerAxes  RotationSequence=XYX  RotationSequenceAngles=[0 0 0]  RotationSequenceAnglesUnits=deg  RotationMatrix=[1 0 0; 0 1 0; 0 0 1]
  Rigid Transform11 : sm_lib/Frames and Transforms/Rigid Transform  TranslationMethod=Cartesian  TranslationStandardOffset=0  TranslationLengthUnit=m  TranslationStandardAxis=+Z  TranslationCartesianOffset=[-DistWorkC*sin(alphaAC) -DistWorkC*cos(alphaAC) 0]  TranslationROffset=0  TranslationROffsetUnits=m  TranslationZOffset=0  TranslationZOffsetUnits=m  TranslationThetaOffset=0  TranslationThetaOffsetUnits=deg  RotationMethod=None  RotationAngleUnits=deg  RotationStandardAxis=+Z  RotationAngle=90  RotationArbitraryAxis=[0 0 1]  FollAlignAxisA=+X  BaseAlignAxisA=+Z  FollAlignAxisB=+Z  BaseAlignAxisB=+X  RotationSequenceAxes=FollowerAxes  RotationSequence=XYX  RotationSequenceAngles=[0 0 0]  RotationSequenceAnglesUnits=deg  RotationMatrix=[1 0 0; 0 1 0; 0 0 1]
  Rigid Transform13 : sm_lib/Frames and Transforms/Rigid Transform  TranslationMethod=None  TranslationStandardOffset=0  TranslationLengthUnit=m  TranslationStandardAxis=+Z  TranslationCartesianOffset=[0 0 0]  TranslationROffset=0  TranslationROffsetUnits=m  TranslationZOffset=0  TranslationZOffsetUnits=m  TranslationThetaOffset=0  TranslationThetaOffsetUnits=deg  RotationMethod=StandardAxis  RotationAngleUnits=rad  RotationStandardAxis=+Y  RotationAngle=(pi/2) + alphaAB  RotationArbitraryAxis=[0 0 1]  FollAlignAxisA=+X  BaseAlignAxisA=+Z  FollAlignAxisB=+Z  BaseAlignAxisB=+X  RotationSequenceAxes=FollowerAxes  RotationSequence=XYX  RotationSequenceAngles=[0 0 0]  RotationSequenceAnglesUnits=deg  RotationMatrix=[1 0 0; 0 1 0; 0 0 1]
  Rigid Transform14 : sm_lib/Frames and Transforms/Rigid Transform  TranslationMethod=Cartesian  TranslationStandardOffset=0  TranslationLengthUnit=m  TranslationStandardAxis=+Z  TranslationCartesianOffset=[-DistWorkB*sin(alphaAB) -DistWorkB*cos(alphaAB) 0]  TranslationROffset=0  TranslationROffsetUnits=m  TranslationZOffset=0  TranslationZOffsetUnits=m  TranslationThetaOffset=0  TranslationThetaOffsetUnits=deg  RotationMethod=None  RotationAngleUnits=deg  RotationStandardAxis=+Z  RotationAngle=90  RotationArbitraryAxis=[0 0 1]  FollAlignAxisA=+X  BaseAlignAxisA=+Z  FollAlignAxisB=+Z  BaseAlignAxisB=+X  RotationSequenceAxes=FollowerAxes  RotationSequence=XYX  RotationSequenceAngles=[0 0 0]  RotationSequenceAnglesUnits=deg  RotationMatrix=[1 0 0; 0 1 0; 0 0 1]
  Rigid Transform16 : sm_lib/Frames and Transforms/Rigid Transform  TranslationMethod=None  TranslationStandardOffset=0  TranslationLengthUnit=m  TranslationStandardAxis=+Z  TranslationCartesianOffset=[0 0 0]  TranslationROffset=0  TranslationROffsetUnits=m  TranslationZOffset=0  TranslationZOffsetUnits=m  TranslationThetaOffset=0  TranslationThetaOffsetUnits=deg  RotationMethod=StandardAxis  RotationAngleUnits=deg  RotationStandardAxis=+Y  RotationAngle=90  RotationArbitraryAxis=[0 0 1]  FollAlignAxisA=+X  BaseAlignAxisA=+Z  FollAlignAxisB=+Z  BaseAlignAxisB=+X  RotationSequenceAxes=FollowerAxes  RotationSequence=XYX  RotationSequenceAngles=[0 0 0]  RotationSequenceAnglesUnits=deg  RotationMatrix=[1 0 0; 0 1 0; 0 0 1]
  Rigid Transform17 : sm_lib/Frames and Transforms/Rigid Transform  TranslationMethod=Cartesian  TranslationStandardOffset=0  TranslationLengthUnit=m  TranslationStandardAxis=+Z  TranslationCartesianOffset=[0 -DistWorkA 0]  TranslationROffset=0  TranslationROffsetUnits=m  TranslationZOffset=0  TranslationZOffsetUnits=m  TranslationThetaOffset=0  TranslationThetaOffsetUnits=deg  RotationMethod=None  RotationAngleUnits=deg  RotationStandardAxis=+Z  RotationAngle=90  RotationArbitraryAxis=[0 0 1]  FollAlignAxisA=+X  BaseAlignAxisA=+Z  FollAlignAxisB=+Z  BaseAlignAxisB=+X  RotationSequenceAxes=FollowerAxes  RotationSequence=XYX  RotationSequenceAngles=[0 0 0]  RotationSequenceAnglesUnits=deg  RotationMatrix=[1 0 0; 0 1 0; 0 0 1]
  Rigid Transform3 : sm_lib/Frames and Transforms/Rigid Transform  TranslationMethod=None  TranslationStandardOffset=0  TranslationLengthUnit=m  TranslationStandardAxis=+Z  TranslationCartesianOffset=[0 0 0]  TranslationROffset=0  TranslationROffsetUnits=m  TranslationZOffset=0  TranslationZOffsetUnits=m  TranslationThetaOffset=0  TranslationThetaOffsetUnits=deg  RotationMethod=StandardAxis  RotationAngleUnits=rad  RotationStandardAxis=+Y  RotationAngle=(pi/2) + alphaAB  RotationArbitraryAxis=[0 0 1]  FollAlignAxisA=+X  BaseAlignAxisA=+Z  FollAlignAxisB=+Z  BaseAlignAxisB=+X  RotationSequenceAxes=FollowerAxes  RotationSequence=XYX  RotationSequenceAngles=[0 0 0]  RotationSequenceAnglesUnits=deg  RotationMatrix=[1 0 0; 0 1 0; 0 0 1]
  Rigid Transform4 : sm_lib/Frames and Transforms/Rigid Transform  TranslationMethod=Cartesian  TranslationStandardOffset=0  TranslationLengthUnit=m  TranslationStandardAxis=+Z  TranslationCartesianOffset=[0;-DistBaseA;0]  TranslationROffset=0  TranslationROffsetUnits=m  TranslationZOffset=0  TranslationZOffsetUnits=m  TranslationThetaOffset=0  TranslationThetaOffsetUnits=deg  RotationMethod=None  RotationAngleUnits=deg  RotationStandardAxis=+Z  RotationAngle=90  RotationArbitraryAxis=[0 0 1]  FollAlignAxisA=+X  BaseAlignAxisA=+Z  FollAlignAxisB=+Z  BaseAlignAxisB=+X  RotationSequenceAxes=FollowerAxes  RotationSequence=XYX  RotationSequenceAngles=[0 0 0]  RotationSequenceAnglesUnits=deg  RotationMatrix=[1 0 0; 0 1 0; 0 0 1]
  Rigid Transform5 : sm_lib/Frames and Transforms/Rigid Transform  TranslationMethod=Cartesian  TranslationStandardOffset=0  TranslationLengthUnit=m  TranslationStandardAxis=+Z  TranslationCartesianOffset=[-DistBaseB*sin(alphaAB) -DistBaseB*cos(alphaAB) 0]  TranslationROffset=0  TranslationROffsetUnits=m  TranslationZOffset=0  TranslationZOffsetUnits=m  TranslationThetaOffset=0  TranslationThetaOffsetUnits=deg  RotationMethod=None  RotationAngleUnits=deg  RotationStandardAxis=+Z  RotationAngle=90  RotationArbitraryAxis=[0 0 1]  FollAlignAxisA=+X  BaseAlignAxisA=+Z  FollAlignAxisB=+Z  BaseAlignAxisB=+X  RotationSequenceAxes=FollowerAxes  RotationSequence=XYX  RotationSequenceAngles=[0 0 0]  RotationSequenceAnglesUnits=deg  RotationMatrix=[1 0 0; 0 1 0; 0 0 1]
  Rigid Transform7 : sm_lib/Frames and Transforms/Rigid Transform  TranslationMethod=None  TranslationStandardOffset=0  TranslationLengthUnit=m  TranslationStandardAxis=+Z  TranslationCartesianOffset=[0 0 0]  TranslationROffset=0  TranslationROffsetUnits=m  TranslationZOffset=0  TranslationZOffsetUnits=m  TranslationThetaOffset=0  TranslationThetaOffsetUnits=deg  RotationMethod=StandardAxis  RotationAngleUnits=rad  RotationStandardAxis=+Y  RotationAngle=(pi/2) + alphaAC  RotationArbitraryAxis=[0 0 1]  FollAlignAxisA=+X  BaseAlignAxisA=+Z  FollAlignAxisB=+Z  BaseAlignAxisB=+X  RotationSequenceAxes=FollowerAxes  RotationSequence=XYX  RotationSequenceAngles=[0 0 0]  RotationSequenceAnglesUnits=deg  RotationMatrix=[1 0 0; 0 1 0; 0 0 1]
  Rigid Transform8 : sm_lib/Frames and Transforms/Rigid Transform  TranslationMethod=Cartesian  TranslationStandardOffset=0  TranslationLengthUnit=m  TranslationStandardAxis=+Z  TranslationCartesianOffset=[-DistBaseC*sin(alphaAC) -DistBaseC*cos(alphaAC) 0]  TranslationROffset=0  TranslationROffsetUnits=m  TranslationZOffset=0  TranslationZOffsetUnits=m  TranslationThetaOffset=0  TranslationThetaOffsetUnits=deg  RotationMethod=None  RotationAngleUnits=deg  RotationStandardAxis=+Z  RotationAngle=90  RotationArbitraryAxis=[0 0 1]  FollAlignAxisA=+X  BaseAlignAxisA=+Z  FollAlignAxisB=+Z  BaseAlignAxisB=+X  RotationSequenceAxes=FollowerAxes  RotationSequence=XYX  RotationSequenceAngles=[0 0 0]  RotationSequenceAnglesUnits=deg  RotationMatrix=[1 0 0; 0 1 0; 0 0 1]
  Simulink-PS Converter : nesl_utility/Simulink-PS Converter  PhysicalDomain=network_engine_domain  SubClassName=ps_input  LeftPortType=input  RightPortType=output  PseudoPeriodic=off  Frequencies=[]  NoiseDistribution=none  NoiseParameters=[]  Unit=rad  AffineConversion=off  FilteringAndDerivatives=filter  SimscapeFilterOrder=2  InputFilterTimeConstant=t_step  UdotUserProvided=0
      settings: SourceProductBaseCode=PW,SS
  Simulink-PS Converter1 : nesl_utility/Simulink-PS Converter  PhysicalDomain=network_engine_domain  SubClassName=ps_input  LeftPortType=input  RightPortType=output  PseudoPeriodic=off  Frequencies=[]  NoiseDistribution=none  NoiseParameters=[]  Unit=rad  AffineConversion=off  FilteringAndDerivatives=filter  SimscapeFilterOrder=2  InputFilterTimeConstant=t_step  UdotUserProvided=0
      settings: SourceProductBaseCode=PW,SS
  Simulink-PS Converter3 : nesl_utility/Simulink-PS Converter  PhysicalDomain=network_engine_domain  SubClassName=ps_input  LeftPortType=input  RightPortType=output  PseudoPeriodic=off  Frequencies=[]  NoiseDistribution=none  NoiseParameters=[]  Unit=rad  AffineConversion=off  FilteringAndDerivatives=filter  SimscapeFilterOrder=2  InputFilterTimeConstant=t_step  UdotUserProvided=0
      settings: SourceProductBaseCode=PW,SS
  Transform Sensor : sm_lib/Frames and Transforms/Transform Sensor  MeasurementFrame=World  SenseAngle=off  SenseAxis=off  SenseAngle1=off  SenseAngle2=off  SenseAngle3=off  SenseQ=off  SenseR=off  SenseOmegaX=off  SenseOmegaY=off  SenseOmegaZ=off  SenseOmega1=off  SenseOmega2=off  SenseOmega3=off  SenseQDot=off  SenseRDot=off  SenseAlphaX=off  SenseAlphaY=off  SenseAlphaZ=off  SenseAlpha1=off  SenseAlpha2=off  SenseAlpha3=off  SenseQDDot=off  SenseRDDot=off  SenseX=on  SenseY=on  SenseZ=on  SenseRad=off  SenseAzim=off  SenseDist=off  SenseInc=off  SenseXDot=on  SenseYDot=on  SenseZDot=on  SenseRadDot=off  SenseAzimDot=off  SenseDistDot=off  SenseIncDot=off  SenseXDDot=on  SenseYDDot=on  SenseZDDot=on  SenseRadDDot=off  SenseAzimDDot=off  SenseDistDDot=off  SenseIncDDot=off
  End Effector Frame : PMIOPort  Side=Right
  Base Frame : PMIOPort  Port=2  Side=Left
  q1 : PMIOPort  Port=3  Side=Right
  dq1 : PMIOPort  Port=4  Side=Right
  ddq1 : PMIOPort  Port=5  Side=Right
  tau1 : PMIOPort  Port=6  Side=Right
  q2 : PMIOPort  Port=7  Side=Right
  dq2 : PMIOPort  Port=8  Side=Right
  ddq2 : PMIOPort  Port=9  Side=Right
  tau2 : PMIOPort  Port=10  Side=Right
  q3 : PMIOPort  Port=11  Side=Right
  dq3 : PMIOPort  Port=12  Side=Right
  ddq3 : PMIOPort  Port=13  Side=Right
  tau3 : PMIOPort  Port=14  Side=Right
  TCP Position : Outport
  TCP Velocity : Outport  Port=2
  TCP Acceleration : Outport  Port=3
  wires:
  PS-Simulink Converter14/1 -> Mux4/1
  PS-Simulink Converter13/1 -> Mux4/3
  Mux4/1 -> TCP Acceleration/1
  PS-Simulink Converter12/1 -> Mux4/2
  PS-Simulink Converter11/1 -> Mux3/3
  PS-Simulink Converter10/1 -> Mux3/2
  Mux3/1 -> TCP Velocity/1
  PS-Simulink Converter9/1 -> Mux3/1
  Mux/1 -> TCP Position/1
  PS-Simulink Converter8/1 -> Mux/3
  PS-Simulink Converter7/1 -> Mux/2
  PS-Simulink Converter6/1 -> Mux/1
  Demux/3 -> Simulink-PS Converter3/1
  Demux/1 -> Simulink-PS Converter/1
  Actuator Position/1 -> Demux/1
  Demux/2 -> Simulink-PS Converter1/1
  connections:
  PS-Simulink Converter13/LConn1 -- Transform Sensor/RConn10
  Transform Sensor/RConn9 -- PS-Simulink Converter12/LConn1
  PS-Simulink Converter14/LConn1 -- Transform Sensor/RConn8
  Transform Sensor/RConn7 -- PS-Simulink Converter11/LConn1
  Transform Sensor/RConn6 -- PS-Simulink Converter10/LConn1
  PS-Simulink Converter9/LConn1 -- Transform Sensor/RConn5
  PS-Simulink Converter8/LConn1 -- Transform Sensor/RConn4
  PS-Simulink Converter7/LConn1 -- Transform Sensor/RConn3
  PS-Simulink Converter6/LConn1 -- Transform Sensor/RConn2
  Rigid Transform16/RConn1 -- Bottom Plate Joint 1/RConn1
  Rigid Transform17/RConn1 -- Rigid Transform15/LConn1
  Rigid Transform15/RConn1 -- Rigid Transform16/LConn1
  Rigid Transform13/RConn1 -- Bottom Plate Joint 2/RConn1
  Rigid Transform12/RConn1 -- Rigid Transform13/LConn1
  Rigid Transform14/RConn1 -- Rigid Transform12/LConn1
  Rigid Transform10/RConn1 -- Bottom Plate Joint 3/RConn1
  Rigid Transform10/LConn1 -- Rigid Transform9/RConn1
  Rigid Transform11/RConn1 -- Rigid Transform9/LConn1
  Rigid Transform7/RConn1 -- Actuator 3/LConn1
  Rigid Transform7/LConn1 -- Rigid Transform6/RConn1
  Rigid Transform8/RConn1 -- Rigid Transform6/LConn1
  Rigid Transform2/RConn1 -- Rigid Transform3/LConn1
  Rigid Transform5/RConn1 -- Rigid Transform2/LConn1
  Rigid Transform/RConn1 -- Rigid Transform1/LConn1
  Rigid Transform3/RConn1 -- Actuator 2/LConn1
  Rigid Transform4/RConn1 -- Rigid Transform/LConn1
  Base Frame/RConn1 -- Transform Sensor/LConn1 -- Base Plate/RConn1 -- Rigid Transform4/LConn1 -- Rigid Transform8/LConn1 -- Rigid Transform5/LConn1
  Actuator 3/LConn2 -- Simulink-PS Converter3/RConn1
  Actuator 2/LConn2 -- Simulink-PS Converter1/RConn1
  Simulink-PS Converter/RConn1 -- Actuator 1/LConn2
  Arm A/RConn1 -- Bottom Plate Joint 1/LConn1
  Arm A/LConn1 -- Actuator 1/RConn1
  Arm B/LConn1 -- Actuator 2/RConn1
  Arm C/LConn1 -- Actuator 3/RConn1
  Arm B/RConn1 -- Bottom Plate Joint 2/LConn1
  Arm C/RConn1 -- Bottom Plate Joint 3/LConn1
  Transform Sensor/RConn1 -- Bottom Plate/RConn1 -- End Effector Frame/RConn1 -- Rigid Transform17/LConn1 -- Rigid Transform14/LConn1 -- Rigid Transform11/LConn1
  Rigid Transform1/RConn1 -- Actuator 1/LConn1
  q1/RConn1 -- Actuator 1/RConn2
  dq1/RConn1 -- Actuator 1/RConn3
  ddq1/RConn1 -- Actuator 1/RConn4
  tau1/RConn1 -- Actuator 1/RConn5
  tau2/RConn1 -- Actuator 2/RConn5
  ddq2/RConn1 -- Actuator 2/RConn4
  dq2/RConn1 -- Actuator 2/RConn3
  Actuator 2/RConn2 -- q2/RConn1
  q3/RConn1 -- Actuator 3/RConn2
  dq3/RConn1 -- Actuator 3/RConn3
  ddq3/RConn1 -- Actuator 3/RConn4
  tau3/RConn1 -- Actuator 3/RConn5
